simulink model "sens_mtr"  (R2022a)
settings: Solver=FixedStepAuto  StartTime=0.0  StopTime=30  RelTol=1e-3  EnableMultiTasking=on
libraries: mbedblockslib x6, hdlsllib x1
settings Model: SimulationMode=external  ExtModeTrigDuration=10  Creator=MATLAB  LastModifiedBy=FUGAZI
settings OptimizationCC: EnhancedBackFolding=on  PassReuseOutputArgsAs=Individual arguments  ZeroExternalMemoryAtStartup=off  ZeroInternalMemoryAtStartup=off  MaxStackSize=64  OptimizeBlockOrder=speed  DifferentSizesBufferReuse=on  OptimizationCustomize=off  EfficientTunableParamExpr=on
settings DebuggingCC: ParameterTunabilityLossMsg=error  UnconnectedInputMsg=warning  UnconnectedOutputMsg=warning  UnconnectedLineMsg=warning
settings HardwareCC: ProdBitPerPointer=32  ProdBitPerSizeT=32  ProdBitPerPtrDiffT=32  ProdLargestAtomicInteger=Long  ProdLargestAtomicFloat=Double  ProdWordSize=32  ProdHWDeviceType=ARM Compatible->ARM Cortex
settings SFSimCC: MATLABDynamicMemAlloc=off
settings RTWCC: SystemTargetFile=ert.tlc  HardwareBoard=STM32 Nucleo L476RG  TemplateMakefile=ert_default_tmf  Toolchain=GNU Tools for ARM Embedded Processors  DLArmComputeVersion=19.05
settings CodeAppCC: ForceParamTrailComments=on  IgnoreCustomStorageClasses=off  OperatorAnnotations=on  SimulinkDataObjDesc=on  SFDataObjDesc=on  InsertBlockDesc=on
settings ERTTargetCC: SupportContinuousTime=on  ExtMode=on  ExtModeTransport=3  ExtModeStaticAlloc=on  ExtModeStaticAllocSize=2000  ExtModeMexFile=ext_xcp  ExtModeMexArgs=1 4 115200  ExtModeIntrfLevel=Level2 - Open

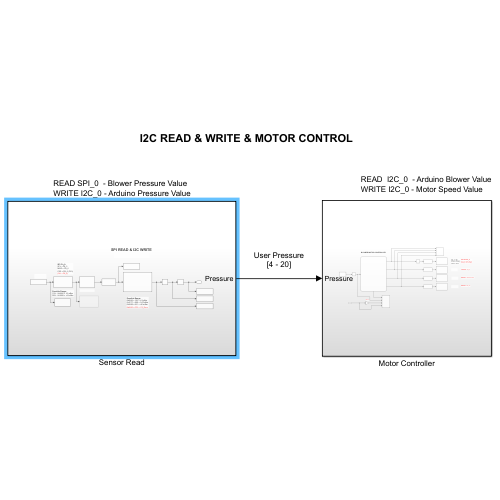
[thumbnail: Simulink's stored preview of the top-level diagram]
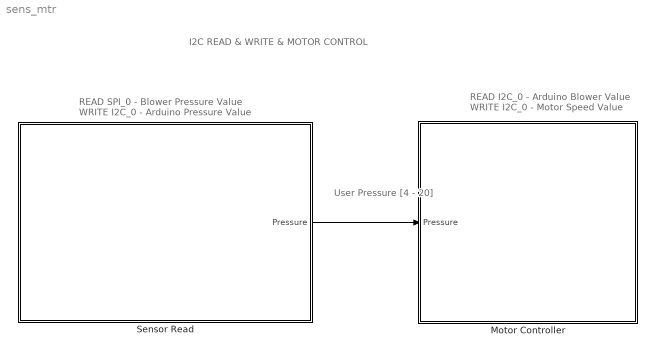
== system sens_mtr ==
  note: User Pressure
      | [4 - 20]
  note: READ SPI_0  - Blower Pressure Value
      | WRITE I2C_0 - Arduino Pressure Value
  note: I2C READ & WRITE & MOTOR CONTROL
  note: READ  I2C_0  - Arduino Blower Value
      | WRITE I2C_0 - Motor Speed Value
  Motor Controller : Subsystem
  Sensor Read : Subsystem
  wires:
  Sensor Read/1(Pressure) -> Motor Controller/1(Pressure)

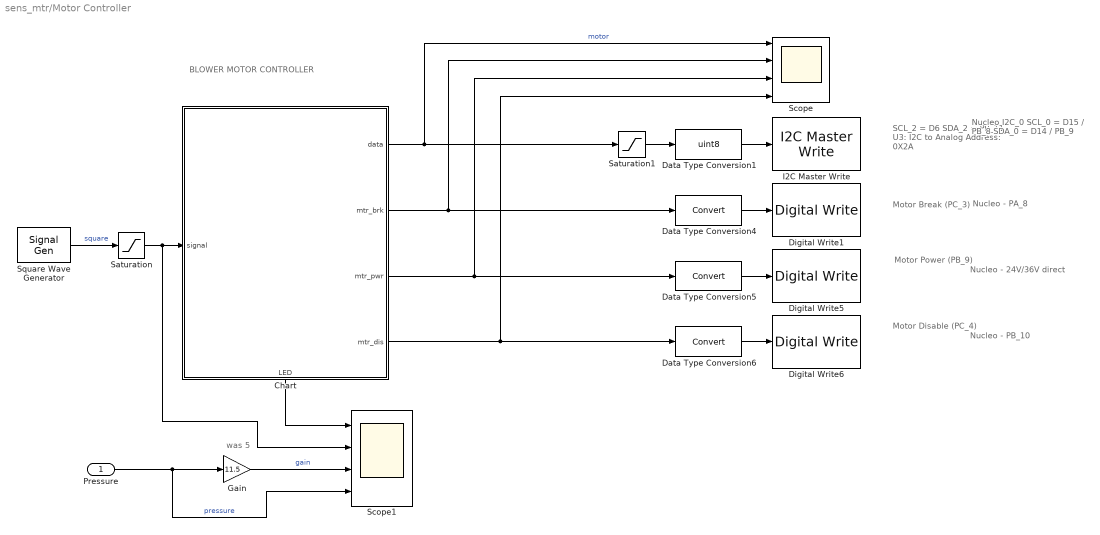
== system sens_mtr/Motor Controller ==
  note: SCL_2 = D6
      | SDA_2 = PB_11
      | U3: I2C to Analog
      | Address: 0X2A
  note: Motor Break
      | (PC_3)
  note: Nucleo - 24V/36V direct
  note: Nucleo - PA_8
  note: Motor Power
      | (PB_9)
  note: Nucleo - PB_10
  note: Motor Disable
      | (PC_4)
  note: Nucleo I2C_0
      | SCL_0 = D15 / PB_8
      | SDA_0 = D14 / PB_9
  note: BLOWER MOTOR CONTROLLER
  note: was 5
  Pressure : Inport
  Chart : Stateflow chart  TreatAsAtomicUnit=on
      settings: PortSchema="{\"entries\":[{\"content\":{\"sides\":[{\"content\":{\"connectorIds\":[\"In1\"]},\"type\":\"ConnectorPlacement.EquallySpacedRectSide\",\"uuid\":\"84df1b4c-bcc9-4224-82b8-1c5b48d4ce5e\"},{\"content\":{\"connectorIds\":[\"Out2\",\"Out3\",\"Out4\",\"Out5\"],\"side\":\"RIGHT\"},\"type\":\"ConnectorPlacement.EquallySpacedRectSide\",\"uuid\":\"0f01030b-4248-47e8-a062-25683a8f3c5c\"},{\"content\":{\"connectorIds\":[],\"side\":\"TOP\"},\"type\":\"ConnectorPlacement.EquallySpacedRectSide\",\"uuid\":\"6351dc8a-8e98-4eac-987b-04ccf0ec8d63\"},{\"content\":{\"connectorIds\":[\"Out1\"],\"side\":\"BOTTOM\"},\"type\":\"ConnectorPlacement.EquallySpacedRectSide\",\"uuid\":\"a1d3854a-5aa8-47eb-a7ef-8ca14fd1287b\"}]},\"type\":\"ConnectorPlacement.EquallySpacedConnector\",\"uuid\":\"a9f2218a-83d6-4a90-85f5-8ad6c25e541e\"}],\"packageUris\":[\"http://schema.mathworks.com/mf0/Connector/R2020b\"],\"version\":\"1.0\"}"
  Data Type Conversion1 : DataTypeConversion  OutDataTypeStr=uint8  SaturateOnIntegerOverflow=off  RndMeth=Floor
  Data Type Conversion4 : DataTypeConversion  SaturateOnIntegerOverflow=off  RndMeth=Floor
  Data Type Conversion5 : DataTypeConversion  SaturateOnIntegerOverflow=off  RndMeth=Floor
  Data Type Conversion6 : DataTypeConversion  SaturateOnIntegerOverflow=off  RndMeth=Floor
  Digital Write1 : mbedblockslib/Digital Write  Pin=PA_8  Direction=output
      settings: SourceProductBaseCode=MICROBIT,NUCLEO,STMICRODIS
  Digital Write5 : mbedblockslib/Digital Write  Pin=PB_5  Direction=output
      settings: SourceProductBaseCode=MICROBIT,NUCLEO,STMICRODIS
  Digital Write6 : mbedblockslib/Digital Write  Pin=PB_10  Direction=output
      settings: SourceProductBaseCode=MICROBIT,NUCLEO,STMICRODIS
  Gain : Gain  Gain=11.5
  I2C Master Write : mbedblockslib/I2C Master Write  I2CModule=0  Mode=Master  SlaveAddress=uint8(hex2dec('2A'))  SlaveByteOrder=BigEndian  Direction=Transmitter  RegisterAddressMode=on  RegisterAddress=uint8(hex2dec('10'))  SlaveDataType=uint8  DataLength=2  NoAck=off  RepeatedStart=off  OutputStatus=off
      settings: SourceProductBaseCode=MICROBIT,NUCLEO,STMICRODIS
  Saturation : Saturate  UpperLimit=250  LowerLimit=15
  Saturation1 : Saturate  UpperLimit=250  LowerLimit=0
  Scope : Scope  NumInputPorts=4
  Scope1 : Scope  NumInputPorts=4
  Square Wave Generator : SignalGenerator  WaveForm=square  Amplitude=100  Units=rad/sec
  wires:
  Data Type Conversion1/1 -> I2C Master Write/1
  Data Type Conversion5/1 -> Digital Write5/1
  Chart/5(mtr_dis) -> Scope/4, Data Type Conversion6/1
  Data Type Conversion4/1 -> Digital Write1/1
  Data Type Conversion6/1 -> Digital Write6/1
  Saturation/1 -> Chart/1(signal), Scope1/2
  Square Wave Generator/1 -> Saturation/1  "square"
  Chart/4(mtr_pwr) -> Scope/3, Data Type Conversion5/1
  Chart/2(data) -> Scope/1, Saturation1/1  "motor"
  Chart/3(mtr_brk) -> Scope/2, Data Type Conversion4/1
  Chart/1(LED) -> Scope1/1
  Pressure/1 -> Scope1/4, Gain/1  "pressure"
  Gain/1 -> Scope1/3  "gain"
  Saturation1/1 -> Data Type Conversion1/1

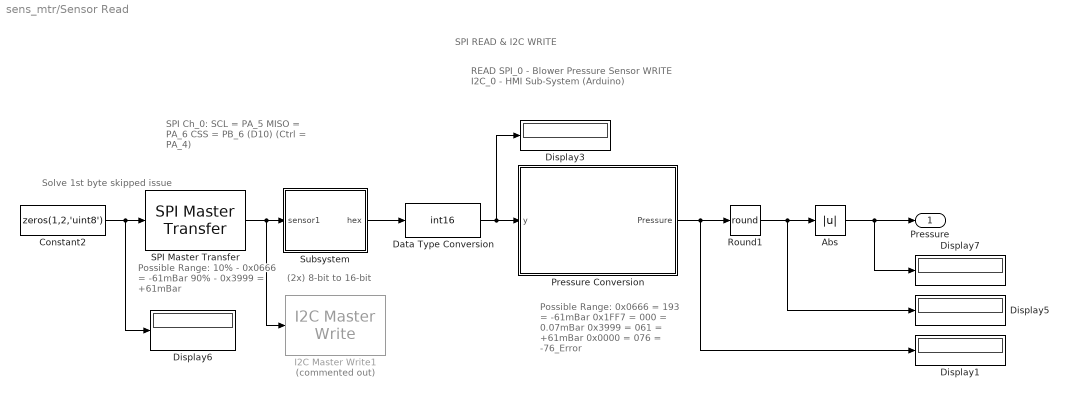
== system sens_mtr/Sensor Read ==
  note: (2x) 8-bit to 16-bit
  note: SPI READ & I2C WRITE
  note: READ SPI_0  -  Blower Pressure Sensor
      | WRITE I2C_0 - HMI Sub-System (Arduino)
  note: SPI Ch_0:
      | SCL = PA_5
      | MISO = PA_6
      | CSS = PB_6 (D10)
      | (Ctrl = PA_4)
  note: Possible Range:
      | 10% - 0x0666 = -61mBar
      | 90% - 0x3999 = +61mBar
  note: Possible Range:
      | 0x0666 = 193 = -61mBar
      | 0x1FF7 = 000 = 0.07mBar
      | 0x3999 = 061 = +61mBar
      | 0x0000 = 076 = -76_Error
  note: Solve 1st byte
      | skipped issue
  Abs : Abs  SaturateOnIntegerOverflow=off
  Constant2 : Constant  Value=zeros(1,2,'uint8')  OutDataTypeStr=uint8
  Data Type Conversion : DataTypeConversion  OutDataTypeStr=int16  SaturateOnIntegerOverflow=off  RndMeth=Floor
  Display{1,3,5..7} (5 alike) : Display
      Display3 settings: Format=hex (Stored Integer)
      Display6 settings: Format=hex (Stored Integer)
  I2C Master Write1 : mbedblockslib/I2C Master Write  Commented=on  I2CModule=0  Mode=Master  SlaveAddress=uint8(hex2dec('55'))  SlaveByteOrder=BigEndian  Direction=Transmitter  RegisterAddressMode=off  RegisterAddress=uint8(hex2dec('11'))  SlaveDataType=uint8  DataLength=2  NoAck=off  RepeatedStart=off  OutputStatus=off
      settings: SourceProductBaseCode=MICROBIT,NUCLEO,STMICRODIS
  Pressure Conversion : Subsystem
  Round1 : Rounding  Operator=round
  SPI Master Transfer : mbedblockslib/SPI Master Transfer  SPIModule=0  Mode=Master  BusSpeed=uint32( 1000000 )  Pin=PB_6  FirstBitToTransfer=Most significant bit (MSB)  ClockMode=0  BlockFunction=Transfer  RegisterAddress=0  OutputDataType=int8  OutputDataLength=1  UseCustomSSPin=Explicit GPIO calls  ActiveLowSSPin=Active low
      settings: SourceProductBaseCode=MICROBIT,NUCLEO,STMICRODIS
  Subsystem : Subsystem
  Pressure : Outport
  wires:
  SPI Master Transfer/1 -> I2C Master Write1/1, Subsystem/1(sensor1)
  Subsystem/1(hex) -> Data Type Conversion/1
  Data Type Conversion/1 -> Display3/1, Pressure Conversion/1(y)
  Pressure Conversion/1(Pressure) -> Display1/1, Round1/1
  Constant2/1 -> Display6/1, SPI Master Transfer/1
  Round1/1 -> Abs/1, Display5/1
  Abs/1 -> Display7/1, Pressure/1

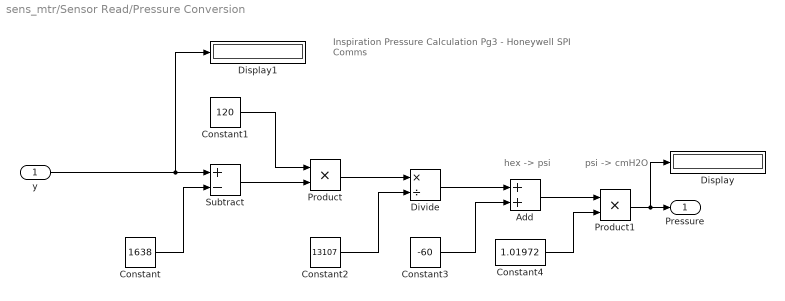
== system sens_mtr/Sensor Read/Pressure Conversion ==
  note: psi -> cmH2O
  note: Inspiration Pressure Calculation
      | Pg3 - Honeywell SPI Comms
  note: hex -> psi
  y : Inport
  Add : Sum
  Constant : Constant  Value=1638
  Constant1 : Constant  Value=120
  Constant2 : Constant  Value=13107
  Constant3 : Constant  Value=-60
  Constant4 : Constant  Value=1.01972
  Display : Display
  Display1 : Display
      settings: Format=hex (Stored Integer)
  Divide : Product  Inputs=*/
  Product : Product
  Product1 : Product
  Subtract : Sum  Inputs=+-
  Pressure : Outport
  wires:
  Constant/1 -> Subtract/2
  Subtract/1 -> Product/2
  Constant1/1 -> Product/1
  Product/1 -> Divide/1
  Constant2/1 -> Divide/2
  Constant3/1 -> Add/2
  Divide/1 -> Add/1
  Add/1 -> Product1/1
  Constant4/1 -> Product1/2
  Product1/1 -> Display/1, Pressure/1
  y/1 -> Display1/1, Subtract/1

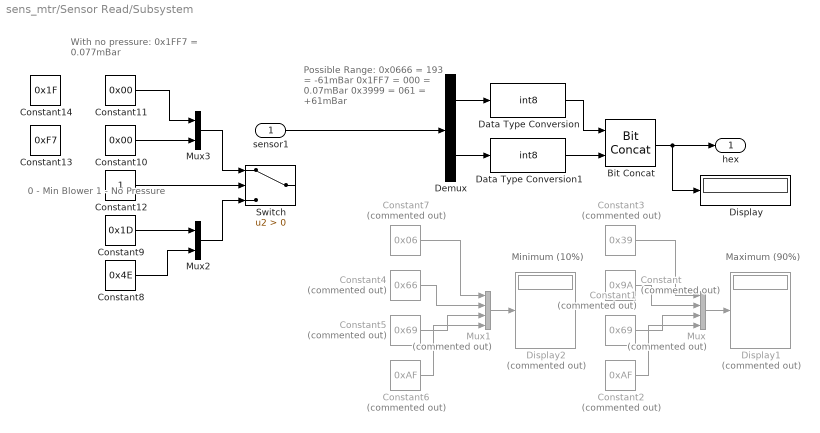
== system sens_mtr/Sensor Read/Subsystem ==
  note: 0 - Min Blower
      | 1 - No Pressure
  note: With no pressure:
      | 0x1FF7 = 0.077mBar
  note: Maximum (90%)
  note: Minimum (10%)
  note: Possible Range:
      | 0x0666 = 193 = -61mBar
      | 0x1FF7 = 000 = 0.07mBar
      | 0x3999 = 061 = +61mBar
  sensor1 : Inport
  Bit Concat : hdlsllib/Logic and Bit Operations/Bit Concat  numInputs=2
  Constant : Constant  Commented=on  Value=0x9A
  Constant1 : Constant  Commented=on  Value=0x69
  Constant10 : Constant  Value=0x00
  Constant11 : Constant  Value=0x00
  Constant12 : Constant
  Constant13 : Constant  Value=0xF7
  Constant14 : Constant  Value=0x1F
  Constant2 : Constant  Commented=on  Value=0xAF
  Constant3 : Constant  Commented=on  Value=0x39
  Constant4 : Constant  Commented=on  Value=0x66
  Constant5 : Constant  Commented=on  Value=0x69
  Constant6 : Constant  Commented=on  Value=0xAF
  Constant7 : Constant  Commented=on  Value=0x06
  Constant8 : Constant  Value=0x4E
  Constant9 : Constant  Value=0x1D
  Data Type Conversion : DataTypeConversion  OutDataTypeStr=int8  SaturateOnIntegerOverflow=off  RndMeth=Floor
  Data Type Conversion1 : DataTypeConversion  OutDataTypeStr=int8  SaturateOnIntegerOverflow=off  RndMeth=Floor
  Demux : Demux  Outputs=2
  Display : Display
      settings: Format=hex (Stored Integer)
  Display1 : Display  Commented=on
      settings: Format=hex (Stored Integer)
  Display2 : Display  Commented=on
      settings: Format=hex (Stored Integer)
  Mux : Mux  Commented=on
  Mux1 : Mux  Commented=on
  Mux2 : Mux  Inputs=2
  Mux3 : Mux  Inputs=2
  Switch : Switch  Criteria=u2 > Threshold  SaturateOnIntegerOverflow=off  InputSameDT=off
  hex : Outport
  wires:
  Constant3/1 -> Mux/1
  Constant/1 -> Mux/2
  Constant1/1 -> Mux/3
  Constant2/1 -> Mux/4
  Data Type Conversion/1 -> Bit Concat/1
  Data Type Conversion1/1 -> Bit Concat/2
  Demux/1 -> Data Type Conversion/1
  Demux/2 -> Data Type Conversion1/1
  Bit Concat/1 -> hex/1, Display/1
  Mux/1 -> Display1/1
  Mux1/1 -> Display2/1
  Constant7/1 -> Mux1/1
  Constant6/1 -> Mux1/4
  Constant5/1 -> Mux1/3
  Constant4/1 -> Mux1/2
  Constant9/1 -> Mux2/1
  Constant8/1 -> Mux2/2
  Constant10/1 -> Mux3/2
  Constant11/1 -> Mux3/1
  Constant12/1 -> Switch/2
  Mux3/1 -> Switch/1
  Mux2/1 -> Switch/3
  sensor1/1 -> Demux/1

== stateflow chart sens_mtr/Motor Controller/Chart ==
  state RUN % Startup Sequence
    state Start_1 % Main Power
      entry:
      mtr_dis = 1; % enabled
      LED = 1; % debug
      exit:
    state Start_2 % Motor Brake
      entry:
      mtr_brk = 1; % Disable
      LED = 0; % debug
      exit:
    state Start_3 % Motor Disable
      entry:
      mtr_pwr = 1; % ON
      LED = 1; % debug
      exit:
    state Start_4 % I2C to Anal.
      entry:
      data = signal; % half spd
      LED = 0; % debug
      exit: %signal = 20;
    (default) -> Start_1 % Main Power
    Start_1 % Main Power -> Start_2 % Motor Brake : after(1,sec)
    Start_2 % Motor Brake -> Start_3 % Motor Disable : after(1,sec)
    Start_3 % Motor Disable -> Start_4 % I2C to Anal. : after(1,sec)
  state Loop % Continuous Update
    state variable_1 % new data
      entry:
      data = signal;
      LED = 1; % debug
      exit:
    state variable_2 % new data
      entry:
      data = signal;
      LED = 0; % debug
      exit:
    (default) -> variable_1 % new data
    variable_2 % new data -> variable_1 % new data : after(3,sec)
    variable_1 % new data -> variable_2 % new data : after(3,sec)
  state SHUTDOWN % Run-Down
    state Stop_1 % I2C to Anal.
      entry:
      data = 0; % slowest?
      LED = 1;
      exit:
    state Stop_2 % Motor Brake
      entry:
      mtr_dis = 0; % slow
      LED = 0; % debug
      exit:
    state Stop_3 % Motor Disable
      entry:
      mtr_brk = 0; % Enable
      LED = 1; % debug
      exit:
    state Stop_4 % Main Power
      entry:
      mtr_pwr = 0; % OFF
      LED = 0; % debug
      exit:
    (default) -> Stop_1 % I2C to Anal.
    Stop_1 % I2C to Anal. -> Stop_2 % Motor Brake : after(2,sec)
    Stop_2 % Motor Brake -> Stop_3 % Motor Disable : after(1,sec)
    Stop_3 % Motor Disable -> Stop_4 % Main Power : after(2,sec)
  note: Power On first
      | then break & disable?
      | or Power after?
  note: What are all of their
      | initial states?
      | (on power up)
  note: BRAKE PIN:
      | Enabled = <0.8V or Gnd
      | Deactivated = >2.4V or Not wired
  note: DISABLE PIN:
      | Disable = <0.8V or Gnd
      | Enable = >2.4V or Not wired
  note: Speed Values:
      | 0xBF = 3/4 Vout
      | 0x7F = 1/2 Vout
      | 0x40 = 1/4 Vout
  note: LOOP BACK TO START-UP
  (default) -> RUN % Startup Sequence
  RUN % Startup Sequence -> Loop % Continuous Update : after(4, sec)
  Loop % Continuous Update -> SHUTDOWN % Run-Down : after(29,sec)
  data: LED output; data output; mtr_brk output; mtr_pwr output; mtr_dis output; signal input
